simulink model "Environment_Simple"  (R2016b)
settings: Solver=VariableStepAuto  StartTime=0.0  StopTime=10.0  RelTol=1e-3
values from neighbouring files (symbols this model uses):
  Env =     [UAV_modelconfig.mat]
libraries: Environment_Lib x1
settings Model: Creator=UAVLAB  LastModifiedBy=UAVLAB

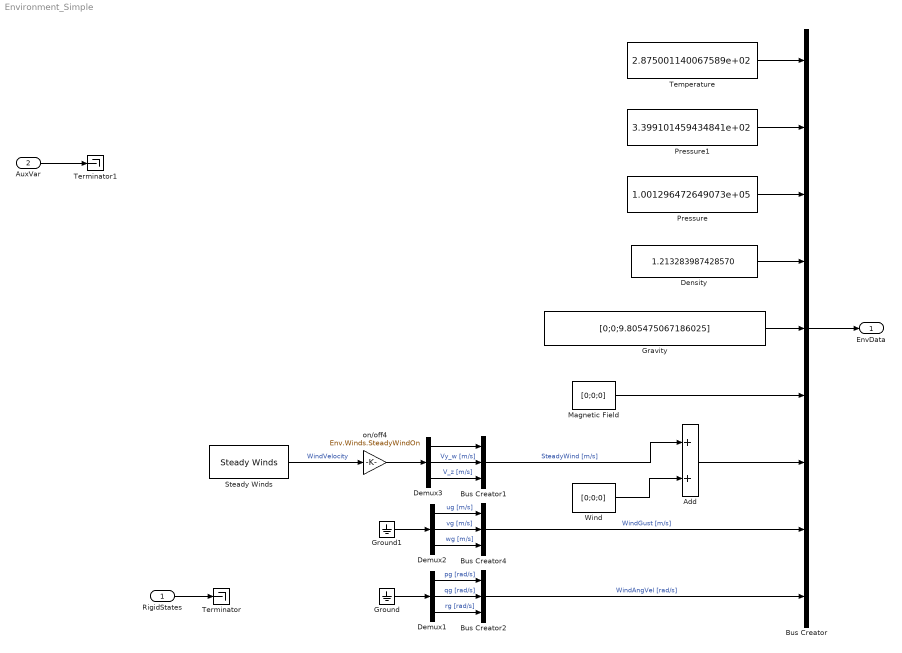
== system Environment_Simple ==
  RigidStates : Inport  OutDataTypeStr=Bus: RigidStates
  AuxVar : Inport  Port=2  OutDataTypeStr=Bus: AuxVar
  Add : Sum
  Bus Creator : BusCreator  Inputs=9  OutDataTypeStr=Bus: EnvData
      settings: InheritFromInputs=off
  Bus Creator1 : BusCreator  Inputs=3
  Bus Creator2 : BusCreator  Inputs=3
  Bus Creator4 : BusCreator  Inputs=3
  Demux1 : Demux  Outputs=3
  Demux2 : Demux  Outputs=3
  Demux3 : Demux  Outputs=3
  Density : Constant  Value=1.213283987428570
  "Gravity " : Constant  Value=[0;0;9.805475067186025]
  Ground : Ground
  Ground1 : Ground
  Magnetic Field : Constant  Value=[0;0;0]
  Pressure : Constant  Value=1.001296472649073e+05
  Pressure1 : Constant  Value=3.399101459434841e+02
  Steady Winds : Environment_Lib/Steady Winds
  Temperature : Constant  Value=2.875001140067589e+02
  Terminator : Terminator
  Terminator1 : Terminator
  Wind : Constant  Value=[0;0;0]
  on/off4 : Gain  Gain=Env.Winds.SteadyWindOn
  EnvData : Outport  OutDataTypeStr=Bus: EnvData
  wires:
  Wind/1 -> Add/2
  RigidStates/1 -> Terminator/1
  Bus Creator/1 -> EnvData/1
  Add/1 -> Bus Creator/7
  Magnetic Field/1 -> Bus Creator/6
  Bus Creator2/1 -> Bus Creator/9  "WindAngVel [rad/s]"
  Bus Creator4/1 -> Bus Creator/8  "WindGust [m/s]"
  Bus Creator1/1 -> Add/1  "SteadyWind [m/s]"
  on/off4/1 -> Demux3/1
  Demux3/2 -> Bus Creator1/2  "Vy_w [m/s]"
  Demux3/3 -> Bus Creator1/3  "V_z [m/s]"
  Ground1/1 -> Demux2/1
  Demux2/2 -> Bus Creator4/2  "vg [m/s]"
  Demux2/3 -> Bus Creator4/3  "wg [m/s]"
  Demux2/1 -> Bus Creator4/1  "ug [m/s]"
  Ground/1 -> Demux1/1
  Steady Winds/1 -> on/off4/1  "WindVelocity"
  Demux1/1 -> Bus Creator2/1  "pg [rad/s]"
  Demux1/2 -> Bus Creator2/2  "qg [rad/s]"
  Demux1/3 -> Bus Creator2/3  "rg [rad/s]"
  Pressure/1 -> Bus Creator/3
  Temperature/1 -> Bus Creator/1
  Pressure1/1 -> Bus Creator/2
  Density/1 -> Bus Creator/4
  "Gravity "/1 -> Bus Creator/5
  AuxVar/1 -> Terminator1/1
  Demux3/1 -> Bus Creator1/1
